simulink model "HCFilter_harness"  (Simulink 7.7)
settings: Solver=FixedStepDiscrete  SolverMode=SingleTasking  StartTime=0.0  StopTime=100  FixedStep=0.1  RelTol=1e-3
InitFcn:
  | if signalbuilder('HCFilter_harness/Signal_Builder','activegroup') == 1
  |   CD_HYD1_FILTER_FUNCTION.DataType = 'uint8';
  |   CD_HYD1_FILTER_FUNCTION.Value = 255;
  | else
  |   CD_HYD1_FILTER_FUNCTION.DataType = 'uint8';
  |   CD_HYD1_FILTER_FUNCTION.Value = 0;
  | end
  | 
  | if signalbuilder('HCFilter_harness/Signal_Builder','activegroup') == 4
  |   CD_HOT_FUNCTION.DataType = 'uint8';
  |   CD_HOT_FUNCTION.Value = 1;
  | else
  |   CD_HOT_FUNCTION.DataType = 'uint8';
  |   CD_HOT_FUNCTION.Value = 0;
  | end
undefined symbols (not defined in the file): ACTIVE, CD_HYD1_FILTER_DEBOUNCE_NORMAL, CD_HYD1_FILTER_DEBOUNCE_NOT_CONNECTED, CD_HYD1_FILTER_DEBOUNCE_PLUGGED, CD_HYD_FILTER_DELAY, COLD, ENGINE_CRANKING, ENGINE_NOT_RUNNING, ENGINE_RUNNING, INACTIVE, NON_FUNCTIONAL, NORMAL, NOT_CONNECTED, PLUGGED, SENDER, sigbuilder_block, srate100
CloseFcn:
  | rtwprivate ssgencode ModelCloseRequest sle_main_controller
settings Model: Creator=smindema  LastModifiedBy=aliebel  CovMetricSettings=dcw  CovCumulativeReport=on  CovModelRefEnable=off
settings MATStruct: SampleTime=0.01  Offset=0  Priority=[1.0]
settings DataIOCC: LimitDataPoints=off  SaveOutput=off  SaveTime=off
settings OptimizationCC: BlockReduction=off  InlineParams=on  ExpressionFolding=off  StateBitsets=on  DataBitsets=on  UseTempVars=on  InitFltsAndDblsToZero=on  NoFixptDivByZeroProtection=on  EfficientFloat2IntCast=on  OptimizeModelRefInitCode=on
settings DebuggingCC: SaveWithParameterizedLinksMsg=none  MultiTaskDSMMsg=warning  MultiTaskCondExecSysMsg=none  IntegerOverflowMsg=none  ModelReferenceCSMismatchMessage=warning
settings HardwareCC: ProdBitPerInt=16  ProdBitPerPointer=16  ProdIntDivRoundTo=Floor  ProdEndianess=BigEndian  ProdWordSize=16  ProdHWDeviceType=Motorola HC12
settings ModelReferenceCC: ModelReferenceNumInstancesAllowed=Single
settings RTWCC: SystemTargetFile=ert.tlc  GenCodeOnly=on  TemplateMakefile=ert_default_tmf  Description=Real-Time Workshop Embedded Coder (no auto configuration)  GenerateReport=on  RetainRTWFile=on  ProcessScript=ert_make_rtw_hook  IncludeHyperlinkInReport=on  LaunchReport=on  IncludeERTFirstTime=on
settings RTWCC: CustomHeaderCode=|
  | #include "cpp_req_defines.h"
  | #include "hw_fin.h"
  | #include "cdata.h"
settings CodeAppCC: IgnoreCustomStorageClasses=off  DefineNamingRule=UpperCase
settings ERTTargetCC: TargetFcnLib=ansi_tfl_tmw.mat  FunctionExecutionProfile=off  MultiwordLength=2048  GenerateSampleERTMain=on  IncludeMdlTerminateFcn=off  SupportAbsoluteTime=off  SupportNonFinite=off  SupportComplex=off  PurelyIntegerCode=on  ERTCustomFileTemplate=gen_rtw_req_defines_h.tlc  GlobalDataDefinition=InSeparateSourceFile  GlobalDataReference=InSeparateHeaderFile  ConvertIfToSwitch=off

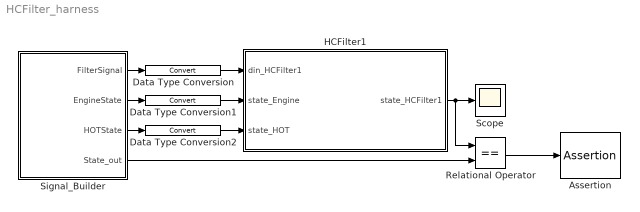
== system HCFilter_harness ==
  Assertion : Assertion  Enabled=off
  Data Type Conversion : DataTypeConversion
  Data Type Conversion1 : DataTypeConversion
  Data Type Conversion2 : DataTypeConversion
  HCFilter1 : Subsystem  TreatAsAtomicUnit=on  SystemSampleTime=srate100  RTWFileName=mod_Inputs
      settings: RTWSystemCode=Function  RTWFileNameOpts=User specified
  Relational Operator : RelationalOperator  Operator===  OutDataTypeStr=boolean
  Scope : Scope
      settings: YMin=8  YMax=8
  Signal_Builder : Subsystem  Tag=STV Subsys  LoadFcn=sigbuilder_block('load',[80.25 256.5 1335.75 422.25 ]);  StartFcn=sigbuilder_block('start');  StopFcn=sigbuilder_block('stop');  ClipboardFcn=sigbuilder_block('clipboard');  mask(Sigbuilder block){}
      mask help: Sigbuilder GUI
      mask init:
      | if ~strcmp(get_param(bdroot(gcbh),'SimulationStatus'),'stopped') tuvar = sigbuilder_block('maskInit'); end
      settings: CopyFcn=sigbuilder_block('copy');  DeleteFcn=sigbuilder_block('delete');  ModelCloseFcn=sigbuilder_block('modelClose');  PreSaveFcn=sigbuilder_block('preSave');  NameChangeFcn=sigbuilder_block('namechange');  OpenFcn=sigbuilder_block('open',[-1200 -225 1200 849.75 ]);  CloseFcn=sigbuilder_block('close');
      mask Display: plot(0,0,100,100,[10,10,40,40,10],[80,20,20,80,80],[40,10],[50,50], [40,27,10],[65,72,56],[40,25,25,10],[28,28,43,43]);
  wires:
  HCFilter1/1(state_HCFilter1) -> Scope/1, Relational Operator/1
  Signal_Builder/1(FilterSignal) -> Data Type Conversion/1
  Signal_Builder/2(EngineState) -> Data Type Conversion1/1
  Signal_Builder/3(HOTState) -> Data Type Conversion2/1
  Data Type Conversion/1 -> HCFilter1/1(din_HCFilter1)
  Data Type Conversion1/1 -> HCFilter1/2(state_Engine)
  Data Type Conversion2/1 -> HCFilter1/3(state_HOT)
  Relational Operator/1 -> Assertion/1
  Signal_Builder/4(State_out) -> Relational Operator/2

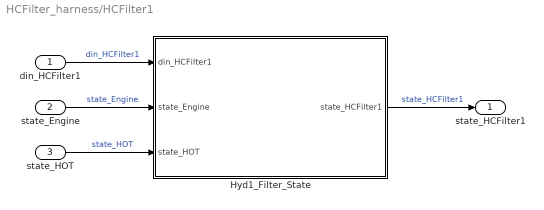
== system HCFilter_harness/HCFilter1 ==
  din_HCFilter1 : Inport  OutDataTypeStr=uint8
  state_Engine : Inport  Port=2  OutDataTypeStr=uint8
  state_HOT : Inport  Port=3  OutDataTypeStr=uint8
  Hyd1_Filter_State : Stateflow chart  TreatAsAtomicUnit=on
  state_HCFilter1 : Outport  OutDataTypeStr=uint8
  wires:
  din_HCFilter1/1 -> Hyd1_Filter_State/1(din_HCFilter1)  "din_HCFilter1"
  state_Engine/1 -> Hyd1_Filter_State/2(state_Engine)  "state_Engine"
  Hyd1_Filter_State/1(state_HCFilter1) -> state_HCFilter1/1  "state_HCFilter1"
  state_HOT/1 -> Hyd1_Filter_State/3(state_HOT)  "state_HOT"

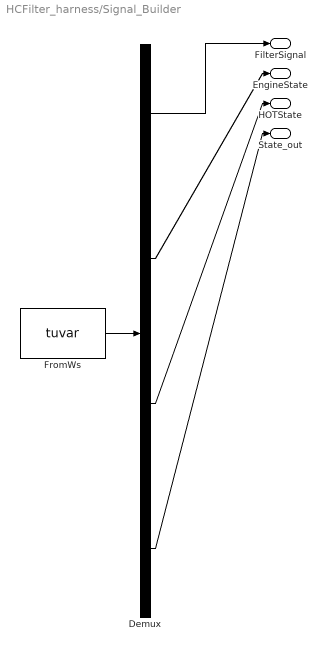
== system HCFilter_harness/Signal_Builder ==
  Demux : Demux  Tag=STV Demux
  FromWs : FromWorkspace  Tag=STV FromWs  VariableName=tuvar  SampleTime=0  SigBuilderData=DataTag0  VnvData=DataTag1
      SigBuilderData=|
      | common.afterFinalStr = 'Extrapolate'
      | common.sampleTime = 0
      | dataSet(1).timeRange = [0 100]
      | dataSet(1).name = 'T1-NONFUNC'
      | dataSet(2).timeRange = [0 100]
      | dataSet(2).name = 'T2-Not Connected'
      | dataSet(3).timeRange = [0 100]
      | dataSet(3).name = 'T3-PLUGGED'
      | dataSet(4).timeRange = [0 100]
      | dataSet(4).name = 'T4-HOT Switch'
      | sbobj.Groups(1).Name = 'T1-NONFUNC'
      | sbobj.Groups(1).Signals(1).Name = 'FilterSignal'
      | sbobj.Groups(1).Signals(1).XData = [0 10 10 11.8 11.8 16 16 19 19 30 30 42.3 42.3 43 43 68 68 69.9 69.9 71 71 74.8 100]
      | sbobj.Groups(1).Signals(1).YData = [0 0 1 1 0 0 1 1 0 0 1 1 0 0 1 1 0 0 1 1 0 0 0]
      | sbobj.Groups(1).Signals(2).Name = 'EngineState'
      | sbobj.Groups(1).Signals(2).XData = [0 15.6 15.6 19.8 19.8 61.2 61.2 72.1 72.1 100]
      | sbobj.Groups(1).Signals(2).YData = [1 1 2 2 1 1 3 3 1 1]
      | sbobj.Groups(1).Signals(3).Name = 'HOTState'
      | sbobj.Groups(1).Signals(3).XData = [0 100]
      | sbobj.Groups(1).Signals(3).YData = [8 8]
      | sbobj.Groups(1).Signals(4).Name = 'State_out'
      | sbobj.Groups(1).Signals(4).XData = [0 100]
      | sbobj.Groups(1).Signals(4).YData = [8 8]
      | sbobj.Groups(2).Name = 'T2-Not Connected'
      | sbobj.Groups(2).Signals(1).Name = 'FilterSignal'
      | sbobj.Groups(2).Signals(1).XData = [0 10 10 10.6 10.6 15.9 15.9 16.4 16.4 33.7 33.7 69.8 69.8 70.3 70.3 88.9 88.9 100]
      | sbobj.Groups(2).Signals(1).YData = [0 0 1 1 0 0 1 1 0 0 1 1 0 0 1 1 0 0]
      | sbobj.Groups(2).Signals(2).Name = 'EngineState'
      | sbobj.Groups(2).Signals(2).XData = [0 12.4 12.4 76.2 76.2 85.4 85.4 100]
      | sbobj.Groups(2).Signals(2).YData = [15 15 1 1 2 2 1 1]
      | sbobj.Groups(2).Signals(3).Name = 'HOTState'
      | sbobj.Groups(2).Signals(3).XData = [0 100]
      | sbobj.Groups(2).Signals(3).YData = [8 8]
      | sbobj.Groups(2).Signals(4).Name = 'State_out'
      | sbobj.Groups(2).Signals(4).XData = [0 63.8 63.8 94 94 100]
      | sbobj.Groups(2).Signals(4).YData = [8 8 16 16 8 8]
      | sbobj.Groups(3).Name = 'T3-PLUGGED'
      | sbobj.Groups(3).Signals(1).Name = 'FilterSignal'
      | sbobj.Groups(3).Signals(1).XData = [0 22.5 33.8 33.8 35.5 35.5 39.3 39.3 39.7 39.7 89.5 89.5 90.1 90.1 94.1 94.1 94.8 94.8 95.5 95.5 100]
      | sbobj.Groups(3).Signals(1).YData = [1 1 1 0 0 1 1 0 0 1 1 0 0 1 1 0 0 1 1 0 0]
      | sbobj.Groups(3).Signals(2).Name = 'EngineState'
      | sbobj.Groups(3).Signals(2).XData = [0 20.1 20.1 40.8 100]
      | sbobj.Groups(3).Signals(2).YData = [1 1 3 3 3]
      | sbobj.Groups(3).Signals(3).Name = 'HOTState'
      | sbobj.Groups(3).Signals(3).XData = [0 27 27 37.4 37.4 43.9 43.9 46.7 46.7 48.2 48.2 100]
      | sbobj.Groups(3).Signals(3).YData = [12 12 8 8 12 12 8 8 12 12 8 8]
      | sbobj.Groups(3).Signals(4).Name = 'State_out'
      | sbobj.Groups(3).Signals(4).XData = [0 30.3 30.3 33.9 33.9 78.3 78.3 100]
      | sbobj.Groups(3).Signals(4).YData = [8 8 16 16 8 8 17 17]
      | sbobj.Groups(4).Name = 'T4-HOT Switch'
      | sbobj.Groups(4).Signals(1).Name = 'FilterSignal'
      | sbobj.Groups(4).Signals(1).XData = [0 8.4 8.4 9.8 9.8 11.3 11.3 16.9 16.9 17.9 17.9 89.5 89.5 90.1 90.1 95.5 95.5 100]
      | sbobj.Groups(4).Signals(1).YData = [0 0 1 1 0 0 1 1 0 0 1 1 0 0 1 1 0 0]
      | sbobj.Groups(4).Signals(2).Name = 'EngineState'
      | sbobj.Groups(4).Signals(2).XData = [0 10.4 10.4 12.5 12.5 15.1 15.1 17.3 17.3 87.2 87.2 91.2 91.2 100]
      | sbobj.Groups(4).Signals(2).YData = [1 1 2 2 3 3 1 1 3 3 1 1 3 3]
      | sbobj.Groups(4).Signals(3).Name = 'HOTState'
      | sbobj.Groups(4).Signals(3).XData = [0 27 32.8 37.5 100]
      | sbobj.Groups(4).Signals(3).YData = [8 8 8 8 8]
      | sbobj.Groups(4).Signals(4).Name = 'State_out'
      | sbobj.Groups(4).Signals(4).XData = [0 100]
      | sbobj.Groups(4).Signals(4).YData = [8 8]
  FilterSignal : Outport  Tag=STV Outport
  EngineState : Outport  Tag=STV Outport  Port=2
  HOTState : Outport  Tag=STV Outport  Port=3
  State_out : Outport  Tag=STV Outport  Port=4
  wires:
  Demux/1 -> FilterSignal/1
  FromWs/1 -> Demux/1
  Demux/2 -> EngineState/1
  Demux/3 -> HOTState/1
  Demux/4 -> State_out/1

== stateflow chart HCFilter1/Hyd1_Filter_State ==
  note: Once we crank we do not want to be able to detecte NOT_CONNECTED again
      | because the system becomes pressurised and with could oil could trip a falase
      | not connected alarm.
  state DEBOUNCE_COLD
    en:debounceCount = 0;
    du:debounceCount++;
    ex:FilterDelay = ACTIVE;
  state PLUGGED
    state PLUGGED
      en:state_HCFilter1 = PLUGGED;
    state DEBOUNCE
      en:debounceCount = 0;
      du:debounceCount++;
    (default) -> DEBOUNCE
    DEBOUNCE -> PLUGGED.PLUGGED : [(debounceCount >= CD_HYD1_FILTER_DEBOUNCE_PLUGGED)]
  state NON_FUNCTIONAL
    en:state_HCFilter1 = NORMAL;
  state NORMAL_AFTER_CRANK
    en:state_HCFilter1 = NORMAL;
  state NOT_CONNECTED
    state NOT_CONNECTED
      en:state_HCFilter1 = NOT_CONNECTED;
    state Debounce
      en:debounceCount = 0;
      du:debounceCount++;
    (default) -> NOT_CONNECTED.Debounce
    NOT_CONNECTED.Debounce -> NOT_CONNECTED.NOT_CONNECTED : [(debounceCount >= CD_HYD1_FILTER_DEBOUNCE_NOT_CONNECTED)...
        | || (state_HCFilter1 == NOT_CONNECTED)]
  state NORMAL_NO_CRANK
    state Debounce
      en:debounceCount = 0;
      du:debounceCount++;
    state NORMAL
      en:state_HCFilter1 = NORMAL;
    NORMAL_NO_CRANK.Debounce -> NORMAL : [(debounceCount >= CD_HYD1_FILTER_DEBOUNCE_NORMAL)...
        | || (state_HCFilter1 == NORMAL)]
    (default) -> NORMAL_NO_CRANK.Debounce
  NORMAL_NO_CRANK -> NORMAL_AFTER_CRANK [order 1] : [(state_Engine == ENGINE_CRANKING)...
      | || (state_Engine == ENGINE_RUNNING)]
  NORMAL_AFTER_CRANK -> PLUGGED [order 2] : [(din_HCFilter1 == ACTIVE)...
      | && (((CD_HOT_FUNCTION == SENDER) && (state_HOT != COLD)) || ((CD_HOT_FUNCTION != SENDER) && (FilterDelay == ACTIVE)))...
      | && (state_Engine == ENGINE_RUNNING)]
  NORMAL_AFTER_CRANK -> DEBOUNCE_COLD [order 1] : [(CD_HOT_FUNCTION != SENDER)...
      | && (state_Engine == ENGINE_RUNNING)...
      | && (FilterDelay == INACTIVE)]
  DEBOUNCE_COLD -> NORMAL_AFTER_CRANK : [(debounceCount >= CD_HYD_FILTER_DELAY)]
  PLUGGED -> NORMAL_AFTER_CRANK : [((din_HCFilter1 == INACTIVE) || (state_HOT == COLD))...
      | && (state_HCFilter1 == NORMAL)]
  (default) -> NON_FUNCTIONAL
  NON_FUNCTIONAL -> NORMAL_NO_CRANK : [(CD_HYD1_FILTER_FUNCTION != NON_FUNCTIONAL)]
  NORMAL_NO_CRANK -> NOT_CONNECTED [order 2] : [(din_HCFilter1 == ACTIVE)...
      | && (state_Engine == ENGINE_NOT_RUNNING)]
  NOT_CONNECTED -> NORMAL_NO_CRANK : [(din_HCFilter1 != ACTIVE)]
  data: din_HCFilter1 input uint8; state_Engine input uint8; state_HCFilter1 output uint8; debounceCount local uint16; CD_HYD1_FILTER_FUNCTION parameter uint8; CD_HYD1_FILTER_DEBOUNCE_NORMAL parameter uint16; CD_HYD1_FILTER_DEBOUNCE_PLUGGED parameter uint16; state_HOT input uint8; CD_HOT_FUNCTION parameter uint8; FilterDelay local uint8 =0; CD_HYD_FILTER_DELAY parameter uint16; ACTIVE parameter uint8 =1; INACTIVE parameter uint8 =0; ENGINE_RUNNING parameter uint8 =3; COLD parameter uint8 =12; PLUGGED parameter uint8 =17; NON_FUNCTIONAL parameter uint8 =255; NORMAL parameter uint8 =8; SENDER parameter uint8 =0; NOT_CONNECTED parameter uint8 =16; ENGINE_NOT_RUNNING parameter uint8 =3; CD_HYD1_FILTER_DEBOUNCE_NOT_CONNECTED parameter uint16; ENGINE_CRANKING parameter uint8 =3
